simulink library "utility_service_lib"  (Simulink 8.1)
settings: Solver=ode45  StartTime=0.0  StopTime=10.0  RelTol=1e-3
undefined symbols (not defined in the file): Left, SUBSTATION, Ts, type, V
libraries: cables_lib x12, rtlab x6, simulink x5, breaker_lib x4, Load_lib x4, relay_modbus_lib x3, rtio_generic_modbus x3, transformer_lib x3, EasyGen3500_GensetSignalScaling_lib x2, Banshee_SEL751_Woodward_lib x1, fault_lib x1, SEL751_SignalScaling_lib x1
settings Model: Creator=RE25624  LastModifiedBy=RE25624

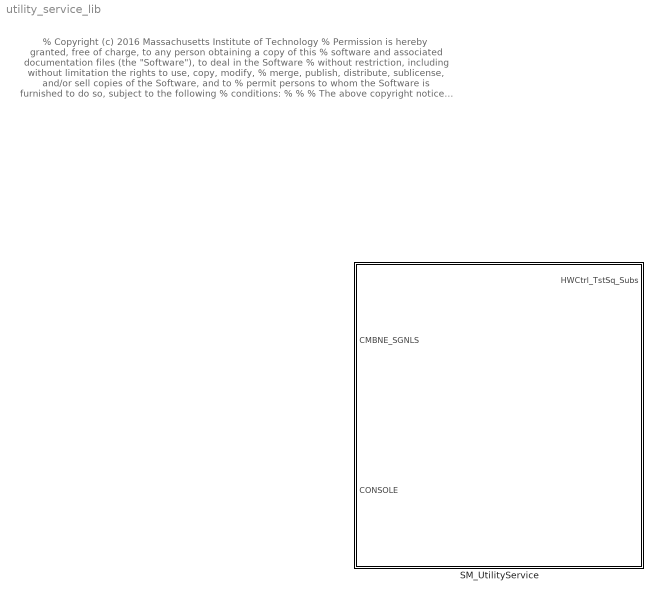
== system utility_service_lib ==
  note: % Copyright (c) 2016 Massachusetts Institute of Technology
      | % Permission is hereby granted, free of charge, to any person obtaining a copy of this
      | % software and associated documentation files (the "Software"), to deal in the Software
      | % without restriction, including without limitation the rights to use, copy, modify,
      | % merge, publish, distribute, sublicense, and/or sell copies of the Software, and to
      | % permit persons to whom the Software is furnished to do so, subject to the following
      | % conditions:
      | %
      | %
      | % The above copyright notice and this permission notice shall be included in
      | % all copies or substantial portions of the Software.
      | %
      | % THE SOFTWARE IS PROVIDED "AS IS", WITHOUT WARRANTY OF ANY KIND, EXPRESS OR IMPLIED,
      | % INCLUDING BUT NOT LIMITED TO THE WARRANTIES OF MERCHANTABILITY, FITNESS FOR A
      | % PARTICULAR PURPOSE AND NONINFRINGEMENT. IN NO EVENT SHALL THE AUTHORS OR COPYRIGHT
      | % HOLDERS BE LIABLE FOR ANY CLAIM, DAMAGES OR OTHER LIABILITY, WHETHER IN AN ACTION
      | % OF CONTRACT, TORT OR OTHERWISE, ARISING FROM, OUT OF OR IN CONNECTION WITH THE
      | % SOFTWARE OR THE USE OR OTHER DEALINGS IN THE SOFTWARE.
      | %
      | %
      | %%
  SM_UtilityService : Subsystem

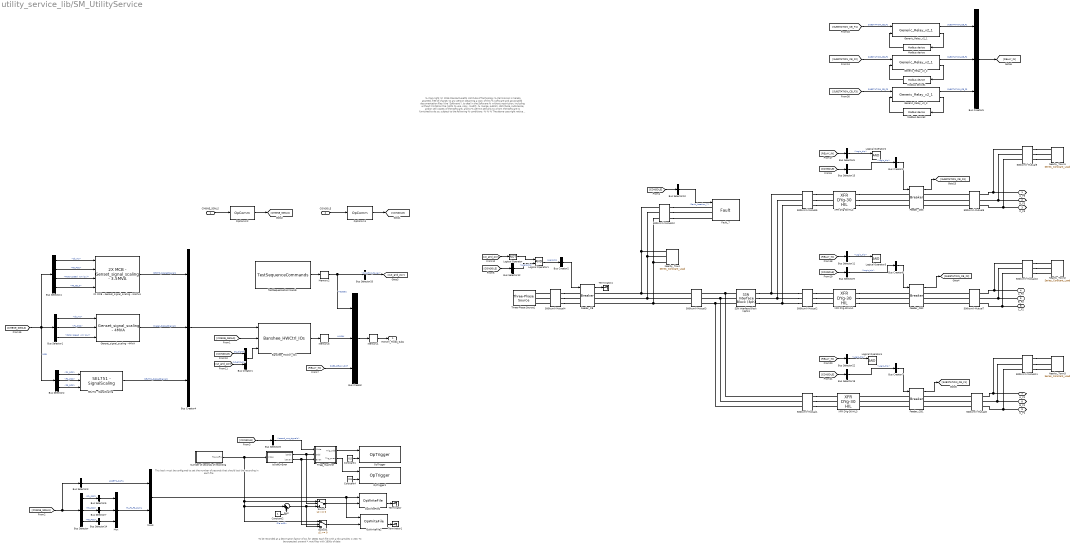
== system utility_service_lib/SM_UtilityService ==
  note: To be recorded at a decimation factor of 10,   for 1800s each file with a Nb samples = 200.
      | To be expected: several *.mat files with 1800s of data
  note: This bock must be configured to set the number of
      | seconds that should last the recording in each file
  note: % Copyright (c) 2016 Massachusetts Institute of Technology
      | % Permission is hereby granted, free of charge, to any person obtaining a copy of this
      | % software and associated documentation files (the "Software"), to deal in the Software
      | % without restriction, including without limitation the rights to use, copy, modify,
      | % merge, publish, distribute, sublicense, and/or sell copies of the Software, and to
      | % permit persons to whom the Software is furnished to do so, subject to the following
      | % conditions:
      | %
      | %
      | % The above copyright notice and this permission notice shall be included in
      | % all copies or substantial portions of the Software.
      | %
      | % THE SOFTWARE IS PROVIDED "AS IS", WITHOUT WARRANTY OF ANY KIND, EXPRESS OR IMPLIED,
      | % INCLUDING BUT NOT LIMITED TO THE WARRANTIES OF MERCHANTABILITY, FITNESS FOR A
      | % PARTICULAR PURPOSE AND NONINFRINGEMENT. IN NO EVENT SHALL THE AUTHORS OR COPYRIGHT
      | % HOLDERS BE LIABLE FOR ANY CLAIM, DAMAGES OR OTHER LIABILITY, WHETHER IN AN ACTION
      | % OF CONTRACT, TORT OR OTHERWISE, ARISING FROM, OUT OF OR IN CONNECTION WITH THE
      | % SOFTWARE OR THE USE OR OTHER DEALINGS IN THE SOFTWARE.
      | %
      | %
      | %%
  CMBNE_SGNLS : Inport
  CONSOLE : Inport  Port=2
  2X MCB - Genset_signal_scaling - 3.5MVA : EasyGen3500_GensetSignalScaling_lib/2X MCB - Genset_signal_scaling - 3.5MVA  Vpk_mcb=11268  watt_mcb=3150000  Vpk_gcb=11268  watt_gcb=3150000  rated_rpm=1800  wm_noise_bias=0.02
  500kcmil-Mutual1 : cables_lib/500kcmil-Mutual  length=200  par_sets=1  ratio=3
  500kcmil-Mutual{3..4,6..11} (8 alike) : cables_lib/500kcmil-Mutual  length=50  par_sets=1  ratio=3
  500kcmil-Mutual12 : cables_lib/500kcmil-Mutual  length=10  par_sets=1  ratio=3
  500kcmil-Mutual2 : cables_lib/500kcmil-Mutual  length=200  par_sets=1  ratio=3
  500kcmil-Mutual5 : cables_lib/500kcmil-Mutual  length=200  par_sets=1  ratio=3
  Banshee_HWCtrl_IOs : Banshee_SEL751_Woodward_lib/Banshee_HWCtrl_IOs  SystemSampleTime=-1
  Bus Creator : BusCreator  Inputs=3
  Bus Creator1 : BusCreator  Inputs=2
  Bus Creator{2..3,6..7} (4 alike) : BusCreator  Inputs=1
  Bus Creator4 : BusCreator  Inputs=3
  Bus Creator5 : BusCreator  Inputs=3
  Bus Selector : BusSelector  OutputSignals=PCC_DATA_OUT.F1_PCC,PCC_DATA_OUT.F2_PCC,PCC_DATA_OUT.F3_PCC
  Bus Selector1 : BusSelector  OutputSignals="F1_MS_IN.DIESEL_DATA.DIESEL_GCB.cb_ms,F1_MS_IN.CB_DATA.F1_PCC,F1_MS_IN.DIESEL_DATA.Gen2_meas.w.w.Rotor speed  wm (pu)"
  Bus Selector10 : BusSelector  OutputSignals=fault_cmd.fault_location_7
  Bus Selector11 : BusSelector  OutputSignals=SUBSTATION_CB_F2.Logic_trip
  Bus Selector12 : BusSelector  OutputSignals=GridStatusCtrl.Substation.Logic_trip
  Bus Selector13 : BusSelector  OutputSignals=GridStatusCtrl.Grid_F3.Logic_trip
  Bus Selector14 : BusSelector  OutputSignals=VRMSLL,Freq,kw,kvar  OutputAsBus=on
  Bus Selector19 : BusSelector  OutputSignals=GridStatusCtrl.Grid_F1.Logic_trip
  Bus Selector2 : BusSelector  OutputSignals=F1_MS_IN.CB_DATA.F1_PCC,F2_MS_IN.CB_DATA.F2_PCC,F3_MS_IN.CB_DATA.F3_PCC
  Bus Selector20 : BusSelector  OutputSignals=Cut_Grid_Power
  Bus Selector22 : BusSelector  OutputSignals=SUBSTATION_CB_F1.Logic_trip
  Bus Selector3 : BusSelector  OutputSignals=F1_MS_IN.DIESEL_DATA.DIESEL_GCB.VRMSLL,F1_MS_IN.DIESEL_DATA.DIESEL_GCB.Freq,F1_MS_IN.DIESEL_DATA.DIESEL_GCB.kw,F1_MS_IN.DIESEL_DATA.DIESEL_GCB.kvar,F3_MS_IN.NG_CHP_DATA.NG_CHP_GCB.VRMSLL,F3_MS_IN.NG_CHP_DATA.NG_CHP_GCB.Freq,F3_MS_IN.NG_CHP_DATA.NG_CHP_GCB.kw,F3_MS_IN.NG_CHP_DATA.NG_CHP_GCB.kvar,BESS_PV.EPC.BESS.BESS_MX1.VRMSLL,BESS_PV.EPC.BESS.BESS_MX1.Freq,BESS_PV.EPC.BESS.BESS_MX1.kw,BESS_PV.EPC.BESS.BESS_MX1.kvar,BESS_PV.EPC.PV.PV_MX1.VRMSLL,BESS_PV.EPC.PV.PV_MX1.Freq,BESS_PV.EPC.PV.PV_MX1.kw,BESS_PV.EPC.PV.PV_MX1.kvar  OutputAsBus=on
  Bus Selector4 : BusSelector  OutputSignals="F3_MS_IN.NG_CHP_DATA.NG_CHP_GCB.cb_ms,F3_MS_IN.CB_DATA.F3_PCC,F3_MS_IN.NG_CHP_DATA.Gen1_meas.w.w.Rotor speed  wm (pu),F3_MS_IN.CB_DATA.F3_CB_3"
  Bus Selector5 : BusSelector  OutputSignals=VRMSLL,Freq,kw,kvar  OutputAsBus=on
  Bus Selector6 : BusSelector  OutputSignals=SUBSTATION_CB_F3.Logic_trip
  Bus Selector7 : BusSelector  OutputSignals=VRMSLL,Freq,kw,kvar  OutputAsBus=on
  Bus Selector8 : BusSelector  OutputSignals=DataLogging.record_rms_signals
  Bus Selector9 : BusSelector  OutputSignals=GridStatusCtrl.Grid_F2.Logic_trip
  Constant1 : Constant  Value=0.5
  Constant2 : Constant
  Constant4 : Constant  Value=0.5
  Fault_7 : fault_lib/Fault  FaultResistance=0.1  GroundResistance=0.01  SnubberResistance=1E6
  Feeder_CB{,1..3} (4 alike) : breaker_lib/Breaker  Ts=Ts  mech_delay=cb_mech_delay
  Generic_Relay_v2_1 : relay_modbus_lib/Generic_Relay_v2_1  Ts=Ts  relay_settings=[SUBSTATION(1,:)]
  Generic_Relay_v2_2 : relay_modbus_lib/Generic_Relay_v2_1  Ts=Ts  relay_settings=[SUBSTATION(2,:)]
  Generic_Relay_v2_3 : relay_modbus_lib/Generic_Relay_v2_1  Ts=Ts  relay_settings=[SUBSTATION(3,:)]
  Genset_signal_scaling - 4MVA : EasyGen3500_GensetSignalScaling_lib/Genset_signal_scaling - 4MVA  Vpk_mcb=11268  watt_mcb=3600000  Vpk_gcb=11268  watt_gcb=3600000  rated_rpm=1800  wm_noise_bias=0.02
  Logical Operator : Logic  Operator=NOT  AllPortsSameDT=off  OutDataTypeStr=boolean
  Logical Operator{1..4} (4 alike) : Logic  AllPortsSameDT=off  OutDataTypeStr=boolean
  Memory1 : Memory
  Memory2 : Memory
  Memory3 : Memory
  Modbus device : rtio_generic_modbus/Modbus device  conf_name=SUBSTATION_relay_cfg1.opal  conf_name_mask=SUBSTATION_relay_cfg1.xls  sample_time=Ts
  Modbus device1 : rtio_generic_modbus/Modbus device  conf_name=SUBSTATION_relay_cfg2.opal  conf_name_mask=SUBSTATION_relay_cfg2.xls  sample_time=Ts
  Modbus device2 : rtio_generic_modbus/Modbus device  conf_name=SUBSTATION_relay_cfg3.opal  conf_name_mask=SUBSTATION_relay_cfg3.xls  sample_time=Ts
  Mux : Mux  Inputs=3
  Mux3 : Mux  Inputs=2
  Nearby_Town : Load_lib/Series_Constant_Load  v=115000  kVA=20E3  pf=0.90
  Nearby_Town1 : Load_lib/Series_Constant_Load  v=13800  kVA=5E3  pf=0.90
  Nearby_Town2 : Load_lib/Series_Constant_Load  v=13800  kVA=5E3  pf=0.90
  Nearby_Town3 : Load_lib/Series_Constant_Load  v=13800  kVA=5E3  pf=0.90
  Number of seconds of recording : Subsystem  mask{time_s=1800}
      mask prompts: time_s "Time in seconds"
      mask help: Set the number of seconds that should last the recording in each file.
  OpComm1 : rtlab/OpComm  nbport=1  groupe_acq=1  subsys_rate=0  st=0  Synchronization=on  Interpolation=on  Threshold=1.0  Missed_Data=off  Sim_Time=off  Samples=off  dynSigOut=off  from_console=1  warning_done=off  writeOpCommFile=off  Offset=off
  OpComm2 : rtlab/OpComm  nbport=1  groupe_acq=1  subsys_rate=0  st=0  Synchronization=on  Interpolation=on  Threshold=1.0  Missed_Data=off  Sim_Time=off  Samples=off  dynSigOut=off  from_console=0  warning_done=off  writeOpCommFile=off  Offset=off
  OpTrigger : rtlab/DataLogging/OpTrigger  Trig_Type=TRIGGER SIGNAL >= TRIGGER LEVEL  Trig_Offset=0  Acq_Group=28
  OpTrigger1 : rtlab/DataLogging/OpTrigger  Trig_Type=TRIGGER SIGNAL >= TRIGGER LEVEL  Trig_Offset=0  Acq_Group=29
  OpWriteFile1 : rtlab/DataLogging/OpWriteFile  Static_File=off  varname=recVar  Filename=A_FILE_RECORDED_o.mat  rtpath='./'  nrtpath='.\'  Acq_Group=28  file_size=150000000  write_offline=off  Sim_Mode=off  Nb_Samples=1000  Buffer_size=0
      settings: Decimation=20
  OpWriteFile2 : rtlab/DataLogging/OpWriteFile  Static_File=off  varname=recVar  Filename=A_FILE_RECORDED_e.mat  rtpath='./'  nrtpath='.\'  Acq_Group=29  file_size=150000000  write_offline=off  Sim_Mode=off  Nb_Samples=1000  Buffer_size=0
      settings: Decimation=20
  SEL751 - SignalScaling : SEL751_SignalScaling_lib/SEL751 - SignalScaling  ct_ratio=1/1250  pt_ratio=1/1800
  SSN Interface Block (3ph)3 : ssn_lib/SSN Interface Block (3ph)  nb_phase=3  nb_port=2  p1_type=V-type(Left)  p2_type=V-type (Right)  p3_type=V-type(Left)  p4_type=V-type(Left)  p5_type=V-type(Left)  p6_type=V-type(Left)  p7_type=V-type(Left)  p8_type=V-type(Left)  p9_type=V-type(Left)  p10_type=V-type(Left)  p11_type=V-type(Left)  p12_type=V-type(Left)  p13_type=V-type(Left)  p14_type=V-type(Left)  p15_type=V-type(Left)  p16_type=V-type(Left)  I_port_shunt_resistance=1e9
  Sum : Sum  Inputs=|++
  Switch : Switch
  Switch1 : Switch
  Terminator : Terminator
  Terminator1 : Terminator
  Terminator4 : Terminator
  TestSequenceCommands : TestSeq_slave_lib/TestSequenceCommands
  Three-Phase Source1 : powerlib/Electrical Sources/Three-Phase Source  Voltage=115000 * 1.02  PhaseAngle=0  Frequency=60  InternalConnection=Yg  SpecifyImpedance=on  Resistance=0.8929  Inductance=16.58e-3  ShortCircuitLevel=2000e6  BaseVoltage=115000 * 1.02  XRratio=100  BusType=swing  Pref=0  Qref=0  Qmin=-inf  Qmax=inf
  Trigg_machine : Subsystem
  XFR DYg-30 HIL1 : transformer_lib/XFR DYg-30 HIL  Rating=50000  Vp=115000  Vs=13800  Z=6  XR=30
  XFR DYg-30 HIL2 : transformer_lib/XFR DYg-30 HIL  Rating=50000  Vp=115000  Vs=13800  Z=6  XR=30
  XFR DYg-30 HIL3 : transformer_lib/XFR DYg-30 HIL  Rating=50000  Vp=115000  Vs=13800  Z=6  XR=30
  isOddOrEven : Subsystem
  A_F3 : PMIOPort  Port=1  Side=Right
  B_F3 : PMIOPort  Port=2  Side=Right
  C_F3 : PMIOPort  Port=3  Side=Right
  A_F2 : PMIOPort  Port=4  Side=Right
  B_F2 : PMIOPort  Port=5  Side=Right
  C_F2 : PMIOPort  Port=6  Side=Right
  A_F1 : PMIOPort  Port=7  Side=Right
  B_F1 : PMIOPort  Port=8  Side=Right
  C_F1 : PMIOPort  Port=9  Side=Right
  HWCtrl_TstSq_Subs : Outport
  wires:
  [RELAY_IN] -> Bus Creator/3  "SUBS_RELAY_OUT"
  Bus Selector10/1 -> Fault_7/1  "<fault_location_7>"
  [CONSOLE] -> Bus Selector10/1
  Bus Selector14/1 -> Mux/3
  Bus Selector5/1 -> Mux/1
  Bus Selector7/1 -> Mux/2
  Bus Selector/2 -> Bus Selector7/1  "<F2_PCC>"
  Bus Selector/1 -> Bus Selector5/1  "<F1_PCC>"
  Bus Selector/3 -> Bus Selector14/1  "<F3_PCC>"
  Bus Creator7/1 -> Feeder_CB1/1
  Bus Selector19/1 -> Bus Creator7/1  "<Logic_trip>"
  Bus Selector22/1 -> Logical Operator4/1  "<Logic_trip>"
  [RELAY_IN] -> Bus Selector22/1
  [CONSOLE] -> Bus Selector19/1
  Bus Creator6/1 -> Feeder_CB2/1
  Bus Selector9/1 -> Bus Creator6/1  "<Logic_trip>"
  Bus Selector11/1 -> Logical Operator3/1  "<Logic_trip>"
  [RELAY_IN] -> Bus Selector11/1
  [CONSOLE] -> Bus Selector9/1
  Bus Creator3/1 -> Feeder_CB3/1
  Bus Selector13/1 -> Bus Creator3/1  "<Logic_trip>"
  Bus Selector6/1 -> Logical Operator2/1  "<Logic_trip>"
  [RELAY_IN] -> Bus Selector6/1
  [SUBSTATION_CB_F1] -> Generic_Relay_v2_1/1  "SUBSTATION_CB_F1"
  [SUBSTATION_CB_F2] -> Generic_Relay_v2_2/1  "SUBSTATION_CB_F2"
  [SUBSTATION_CB_F3] -> Generic_Relay_v2_3/1  "SUBSTATION_CB_F3"
  Bus Creator5/1 -> [RELAY_IN]
  Generic_Relay_v2_3/1 -> Bus Creator5/3  "SUBSTATION_CB_F3"
  Generic_Relay_v2_2/1 -> Bus Creator5/2  "SUBSTATION_CB_F2"
  Generic_Relay_v2_1/1 -> Bus Creator5/1  "SUBSTATION_CB_F1"
  Generic_Relay_v2_3/2 -> Modbus device2/1
  Modbus device2/1 -> Generic_Relay_v2_3/2
  Modbus device1/1 -> Generic_Relay_v2_2/2
  Generic_Relay_v2_2/2 -> Modbus device1/1
  Modbus device/1 -> Generic_Relay_v2_1/2
  Generic_Relay_v2_1/2 -> Modbus device/1
  Feeder_CB1/1 -> [SUBSTATION_CB_F1]
  Feeder_CB2/1 -> [SUBSTATION_CB_F2]
  Bus Creator2/1 -> Feeder_CB/1
  Logical Operator1/1 -> Bus Creator2/1  "Logic_trip"
  Logical Operator/1 -> Logical Operator1/1
  [cut_grid_pwr] -> Logical Operator/1
  [cut_grid_pwr] -> Bus Creator1/2  "cut_grid_pwr"
  Bus Selector20/1 -> [cut_grid_pwr]  "<Cut_Grid_Power>"
  Bus Creator1/1 -> Banshee_HWCtrl_IOs/3
  Bus Creator/1 -> Memory1/1
  Memory2/1 -> Bus Selector20/1, Bus Creator/1  "TestSeq"
  Memory3/1 -> Bus Creator/2  "HWCtrl"
  TestSequenceCommands/1 -> Memory2/1
  Banshee_HWCtrl_IOs/1 -> Memory3/1
  Memory1/1 -> HWCtrl_TstSq_Subs/1
  [CONSOLE] -> Bus Creator1/1  "SC_Signal"
  Bus Selector12/1 -> Logical Operator1/2  "<Logic_trip>"
  Feeder_CB3/1 -> [SUBSTATION_CB_F3]
  [CONSOLE] -> Bus Selector13/1
  [CONSOLE] -> Bus Selector12/1
  Feeder_CB/1 -> Terminator4/1
  [CMBNE_SGNLS] -> Bus Selector/1, Bus Selector3/1
  [CONSOLE] -> Bus Selector8/1
  OpComm1/1 -> [CONSOLE]
  CONSOLE/1 -> OpComm1/1
  Mux/1 -> Mux3/2  "F1_F2_F3_DATA"
  Bus Selector3/1 -> Mux3/1  "ASSETS_DATA"
  OpWriteFile2/2 -> Terminator1/1
  OpWriteFile1/2 -> Terminator/1
  Bus Selector8/1 -> Trigg_machine/1(Write)  "<record_rms_signals>"
  Number of seconds of recording/1(file suffix) -> isOddOrEven/1(Index), Sum/1, Switch1/1, Switch/1  "File suffix"
  Sum/1 -> Switch/3, Switch1/3
  Constant2/1 -> Sum/2
  Switch1/1 -> OpWriteFile2/2
  Switch/1 -> OpWriteFile1/2
  isOddOrEven/2(isEven) -> Switch1/2, Trigg_machine/3(Even)
  isOddOrEven/1(isOdd) -> Switch/2, Trigg_machine/2(Odd)
  Constant4/1 -> OpTrigger1/2
  Constant1/1 -> OpTrigger/2
  Trigg_machine/2(Trig_even) -> OpTrigger1/1
  Trigg_machine/1(Trig_odd) -> OpTrigger/1
  Mux3/1 -> OpWriteFile1/1, OpWriteFile2/1
  [CMBNE_SGNLS] -> Banshee_HWCtrl_IOs/2
  Bus Selector4/4 -> 2X MCB - Genset_signal_scaling - 3.5MVA/4  "<F3_CB_3>"
  Bus Selector2/3 -> SEL751 - SignalScaling/3  "<F3_PCC>"
  Bus Selector2/1 -> SEL751 - SignalScaling/1  "<F1_PCC>"
  Bus Selector2/2 -> SEL751 - SignalScaling/2  "<F2_PCC>"
  SEL751 - SignalScaling/1 -> Bus Creator4/3  "SEL751_ScaledSignals"
  OpComm2/1 -> [CMBNE_SGNLS]
  CMBNE_SGNLS/1 -> OpComm2/1
  Bus Selector1/1 -> Genset_signal_scaling - 4MVA/1  "<cb_ms>"
  Bus Selector1/2 -> Genset_signal_scaling - 4MVA/2  "<F1_PCC>"
  Bus Selector1/3 -> Genset_signal_scaling - 4MVA/3  "<Rotor speed  wm (pu)>"
  Bus Creator4/1 -> Banshee_HWCtrl_IOs/1
  Bus Selector4/1 -> 2X MCB - Genset_signal_scaling - 3.5MVA/1  "<cb_ms>"
  Bus Selector4/2 -> 2X MCB - Genset_signal_scaling - 3.5MVA/2  "<F3_PCC>"
  Bus Selector4/3 -> 2X MCB - Genset_signal_scaling - 3.5MVA/3  "<Rotor speed  wm (pu)>"
  [CMBNE_SGNLS] -> Bus Selector1/1, Bus Selector2/1, Bus Selector4/1  "MCB"
  Genset_signal_scaling - 4MVA/1 -> Bus Creator4/2  "Diesel_ScaledSignals"
  2X MCB - Genset_signal_scaling - 3.5MVA/1 -> Bus Creator4/1  "NGCHP_ScaledSignals"
  connections:
  500kcmil-Mutual12/RConn2 -- Fault_7/LConn2
  500kcmil-Mutual12/RConn3 -- Fault_7/LConn3
  500kcmil-Mutual12/RConn1 -- Fault_7/LConn1
  500kcmil-Mutual11/RConn1 -- Nearby_Town3/LConn1
  500kcmil-Mutual11/RConn3 -- Nearby_Town3/LConn3
  500kcmil-Mutual11/RConn2 -- Nearby_Town3/LConn2
  500kcmil-Mutual10/RConn1 -- Nearby_Town2/LConn1
  500kcmil-Mutual10/RConn3 -- Nearby_Town2/LConn3
  500kcmil-Mutual10/RConn2 -- Nearby_Town2/LConn2
  500kcmil-Mutual9/RConn3 -- Nearby_Town1/LConn3
  500kcmil-Mutual9/RConn1 -- Nearby_Town1/LConn1
  500kcmil-Mutual9/RConn2 -- Nearby_Town1/LConn2
  500kcmil-Mutual9/LConn3 -- 500kcmil-Mutual6/RConn3 -- C_F3/RConn1
  500kcmil-Mutual6/RConn1 -- 500kcmil-Mutual9/LConn1 -- A_F3/RConn1
  500kcmil-Mutual6/RConn2 -- 500kcmil-Mutual9/LConn2 -- B_F3/RConn1
  500kcmil-Mutual7/RConn3 -- 500kcmil-Mutual10/LConn3 -- C_F2/RConn1
  500kcmil-Mutual7/RConn1 -- 500kcmil-Mutual10/LConn1 -- A_F2/RConn1
  500kcmil-Mutual7/RConn2 -- 500kcmil-Mutual10/LConn2 -- B_F2/RConn1
  500kcmil-Mutual8/RConn1 -- 500kcmil-Mutual11/LConn1 -- A_F1/RConn1
  500kcmil-Mutual8/RConn3 -- 500kcmil-Mutual11/LConn3 -- C_F1/RConn1
  500kcmil-Mutual8/RConn2 -- 500kcmil-Mutual11/LConn2 -- B_F1/RConn1
  500kcmil-Mutual8/LConn3 -- Feeder_CB1/RConn3
  500kcmil-Mutual8/LConn2 -- Feeder_CB1/RConn2
  500kcmil-Mutual8/LConn1 -- Feeder_CB1/RConn1
  500kcmil-Mutual7/LConn1 -- Feeder_CB2/RConn1
  500kcmil-Mutual7/LConn3 -- Feeder_CB2/RConn3
  500kcmil-Mutual7/LConn2 -- Feeder_CB2/RConn2
  500kcmil-Mutual6/LConn1 -- Feeder_CB3/RConn1
  500kcmil-Mutual6/LConn3 -- Feeder_CB3/RConn3
  500kcmil-Mutual6/LConn2 -- Feeder_CB3/RConn2
  Feeder_CB1/LConn1 -- XFR DYg-30 HIL3/RConn1
  Feeder_CB1/LConn2 -- XFR DYg-30 HIL3/RConn2
  Feeder_CB1/LConn3 -- XFR DYg-30 HIL3/RConn3
  XFR DYg-30 HIL1/RConn1 -- Feeder_CB2/LConn1
  XFR DYg-30 HIL1/RConn2 -- Feeder_CB2/LConn2
  XFR DYg-30 HIL1/RConn3 -- Feeder_CB2/LConn3
  XFR DYg-30 HIL2/RConn3 -- Feeder_CB3/LConn3
  XFR DYg-30 HIL2/RConn2 -- Feeder_CB3/LConn2
  XFR DYg-30 HIL2/RConn1 -- Feeder_CB3/LConn1
  500kcmil-Mutual2/LConn3 -- 500kcmil-Mutual5/LConn3 -- SSN Interface Block (3ph)3/RConn3
  500kcmil-Mutual2/LConn2 -- 500kcmil-Mutual5/LConn2 -- SSN Interface Block (3ph)3/RConn2
  500kcmil-Mutual2/LConn1 -- 500kcmil-Mutual5/LConn1 -- SSN Interface Block (3ph)3/RConn1
  500kcmil-Mutual1/RConn1 -- XFR DYg-30 HIL3/LConn1
  500kcmil-Mutual1/RConn2 -- XFR DYg-30 HIL3/LConn2
  500kcmil-Mutual1/RConn3 -- XFR DYg-30 HIL3/LConn3
  500kcmil-Mutual5/RConn3 -- XFR DYg-30 HIL2/LConn3
  500kcmil-Mutual5/RConn1 -- XFR DYg-30 HIL2/LConn1
  500kcmil-Mutual5/RConn2 -- XFR DYg-30 HIL2/LConn2
  500kcmil-Mutual2/RConn3 -- XFR DYg-30 HIL1/LConn3
  500kcmil-Mutual2/RConn1 -- XFR DYg-30 HIL1/LConn1
  500kcmil-Mutual2/RConn2 -- XFR DYg-30 HIL1/LConn2
  500kcmil-Mutual4/LConn2 -- Three-Phase Source1/RConn2
  500kcmil-Mutual4/LConn1 -- Three-Phase Source1/RConn1
  500kcmil-Mutual4/LConn3 -- Three-Phase Source1/RConn3
  500kcmil-Mutual4/RConn1 -- Feeder_CB/LConn1
  500kcmil-Mutual4/RConn2 -- Feeder_CB/LConn2
  500kcmil-Mutual4/RConn3 -- Feeder_CB/LConn3
  500kcmil-Mutual3/RConn3 -- 500kcmil-Mutual1/LConn3 -- SSN Interface Block (3ph)3/LConn3
  500kcmil-Mutual3/RConn1 -- 500kcmil-Mutual1/LConn1 -- SSN Interface Block (3ph)3/LConn1
  500kcmil-Mutual3/RConn2 -- 500kcmil-Mutual1/LConn2 -- SSN Interface Block (3ph)3/LConn2
  Feeder_CB/RConn2 -- Nearby_Town/LConn2 -- 500kcmil-Mutual12/LConn2 -- 500kcmil-Mutual3/LConn2
  Feeder_CB/RConn1 -- 500kcmil-Mutual12/LConn1 -- Nearby_Town/LConn1 -- 500kcmil-Mutual3/LConn1
  Feeder_CB/RConn3 -- Nearby_Town/LConn3 -- 500kcmil-Mutual12/LConn3 -- 500kcmil-Mutual3/LConn3

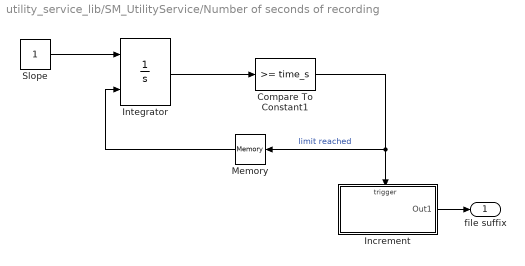
== system utility_service_lib/SM_UtilityService/Number of seconds of recording ==
  Compare To Constant1 : simulink/Logic and Bit Operations/Compare To Constant  relop=>=  const=time_s  OutDataTypeStr=boolean
  Increment : Subsystem
  Integrator : Integrator  ExternalReset=rising
  Memory : Memory
  Slope : Constant
  file suffix : Outport
  wires:
  Slope/1 -> Integrator/1
  Integrator/1 -> Compare To Constant1/1
  Compare To Constant1/1 -> Memory/1, Increment/Trigger  "limit reached"
  Memory/1 -> Integrator/2
  Increment/1(Out1) -> file suffix/1

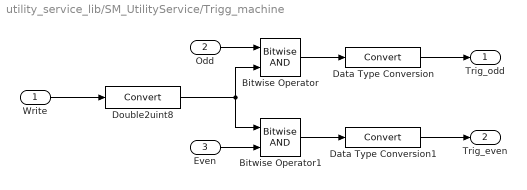
== system utility_service_lib/SM_UtilityService/Trigg_machine ==
  Write : Inport
  Odd : Inport  Port=2
  Even : Inport  Port=3
  Bitwise Operator : simulink/Logic and Bit Operations/Bitwise Operator  logicop=AND  UseBitMask=off  NumInputPorts=2  BitMask=bin2dec('11011001')  BitMaskRealWorld=Stored Integer
  Bitwise Operator1 : simulink/Logic and Bit Operations/Bitwise Operator  logicop=AND  UseBitMask=off  NumInputPorts=2  BitMask=bin2dec('11011001')  BitMaskRealWorld=Stored Integer
  Data Type Conversion : DataTypeConversion
  Data Type Conversion1 : DataTypeConversion
  Double2uint8 : DataTypeConversion
  Trig_odd : Outport
  Trig_even : Outport  Port=2
  wires:
  Double2uint8/1 -> Bitwise Operator1/1, Bitwise Operator/2
  Write/1 -> Double2uint8/1
  Odd/1 -> Bitwise Operator/1
  Data Type Conversion1/1 -> Trig_even/1
  Data Type Conversion/1 -> Trig_odd/1
  Even/1 -> Bitwise Operator1/2
  Bitwise Operator1/1 -> Data Type Conversion1/1
  Bitwise Operator/1 -> Data Type Conversion/1

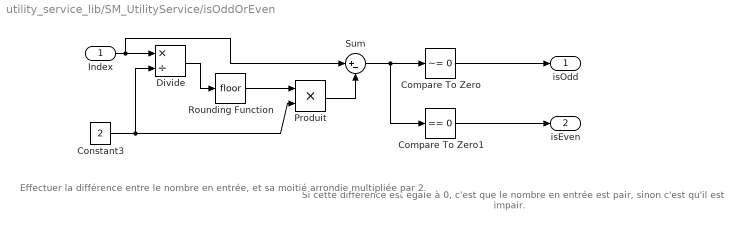
== system utility_service_lib/SM_UtilityService/isOddOrEven ==
  note: Si cette différence est égale à 0, c'est que le
      | nombre en entrée est pair, sinon c'est qu'il est impair.
  note: Effectuer la différence entre le nombre en entrée,
      | et sa moitié arrondie multipliée par 2.
  Index : Inport
  Compare To Zero : simulink/Logic and Bit Operations/Compare To Zero  relop=~=  OutDataTypeStr=boolean  ZeroCross=off
  Compare To Zero1 : simulink/Logic and Bit Operations/Compare To Zero  relop===  OutDataTypeStr=boolean  ZeroCross=off
  Constant3 : Constant  Value=2
  Divide : Product  Inputs=*/  OutDataTypeStr=double
  Produit : Product  Inputs=**  OutDataTypeStr=double
  Rounding Function : Rounding
  Sum : Sum  Inputs=|+-
  isOdd : Outport
  isEven : Outport  Port=2
  wires:
  Compare To Zero1/1 -> isEven/1
  Compare To Zero/1 -> isOdd/1
  Sum/1 -> Compare To Zero1/1, Compare To Zero/1
  Produit/1 -> Sum/2
  Rounding Function/1 -> Produit/1
  Index/1 -> Sum/1, Divide/1
  Divide/1 -> Rounding Function/1
  Constant3/1 -> Produit/2, Divide/2

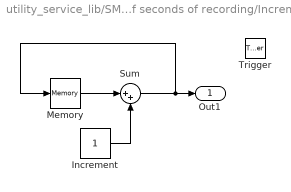
== system utility_service_lib/SM_UtilityService/Number of seconds of recording/Increment ==
  Trigger : TriggerPort
  Increment : Constant
  Memory : Memory  InheritSampleTime=on
  Sum : Sum  Inputs=|++
  Out1 : Outport
  wires:
  Sum/1 -> Out1/1, Memory/1
  Memory/1 -> Sum/1
  Increment/1 -> Sum/2
